simulink model "PI_Model"  (R2020a)
settings: Solver=VariableStepAuto  StartTime=0.0  StopTime=10.0  RelTol=1e-3
PostLoadFcn:
  | a = 3;
  | b = 4;
  | Kp = 36;
  | Ki = 4;
  | m = 25;
  | t = [0:0.01:10]';
  | Ts = 0.01;
  | stin = [zeros(floor((length(t)/2)+1),1) ; 5*ones(floor(length(t)/2),1)];
settings Model: Creator=NIKITA  LastModifiedBy=NIKITA
settings DataIOCC: ExternalInput=[t,stin]  LoadExternalInput=on  SaveFormat=Array  ReturnWorkspaceOutputs=off

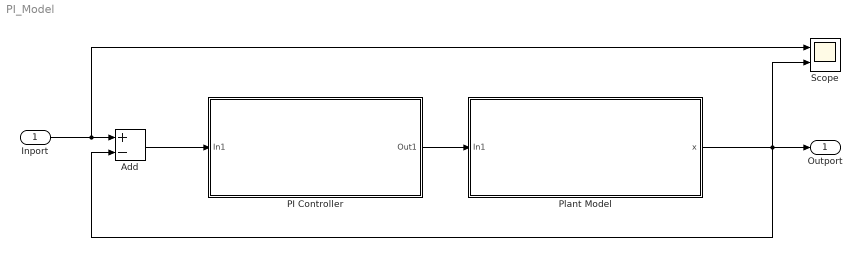
== system PI_Model ==
  Inport : Inport
  Add : Sum  Inputs=+-
  PI Controller : Subsystem
  Plant Model : Subsystem
  Scope : Scope  NumInputPorts=2
  Outport : Outport
  wires:
  PI Controller/1(Out1) -> Plant Model/1(In1)
  Add/1 -> PI Controller/1(In1)
  Inport/1 -> Scope/1, Add/1
  Plant Model/1(x) -> Scope/2, Outport/1, Add/2

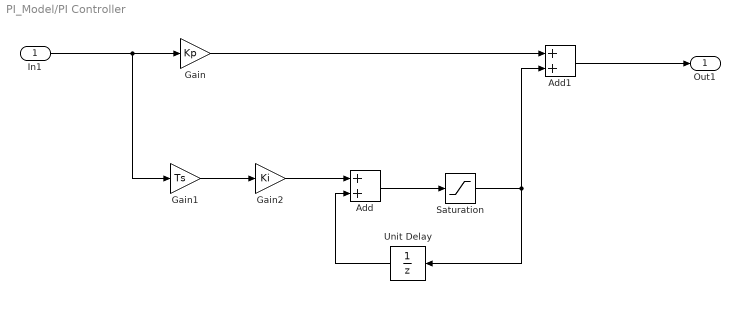
== system PI_Model/PI Controller ==
  In1 : Inport
  Add : Sum
  Add1 : Sum
  Gain : Gain  Gain=Kp
  Gain1 : Gain  Gain=Ts
  Gain2 : Gain  Gain=Ki
  Saturation : Saturate  UpperLimit=1  LowerLimit=-1
  Unit Delay : UnitDelay  SampleTime=-1  HasFrameUpgradeWarning=on
  Out1 : Outport
  wires:
  In1/1 -> Gain1/1, Gain/1
  Add/1 -> Saturation/1
  Saturation/1 -> Unit Delay/1, Add1/2
  Gain1/1 -> Gain2/1
  Gain/1 -> Add1/1
  Unit Delay/1 -> Add/2
  Add1/1 -> Out1/1
  Gain2/1 -> Add/1

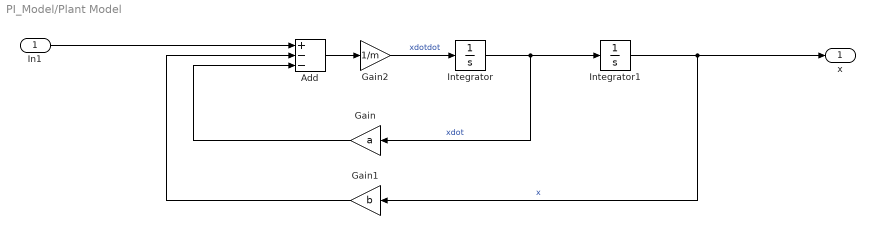
== system PI_Model/Plant Model ==
  In1 : Inport
  Add : Sum  Inputs=+--
  Gain : Gain  Gain=a
  Gain1 : Gain  Gain=b
  Gain2 : Gain  Gain=1/m
  Integrator : Integrator
  Integrator1 : Integrator
  x : Outport
  wires:
  Add/1 -> Gain2/1
  Integrator1/1 -> x/1, Gain1/1  "x"
  Gain1/1 -> Add/2
  Integrator/1 -> Gain/1, Integrator1/1  "xdot"
  Gain2/1 -> Integrator/1  "xdotdot"
  Gain/1 -> Add/3
  In1/1 -> Add/1
